simulink model "ssae_model"  (Simulink 7.3)
settings: Solver=ode3  StartTime=0.0  StopTime=2000.0  FixedStep=1  MaxStep=1  RelTol=1e-3
settings Model: Creator=alkis  LastModifiedBy=alkis
settings DataIOCC: MaxDataPoints=10000
settings DebuggingCC: SolverPrmCheckMsg=none

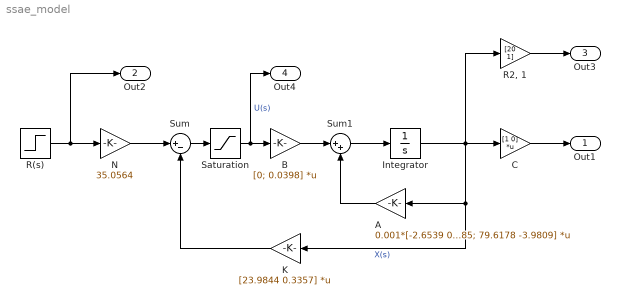
== system ssae_model ==
  A : Gain  Gain=0.001*[-2.6539 0.0885; 79.6178 -3.9809]  Multiplication=Matrix(K*u)  ParameterDataType=fixdt(1, 16)  ParameterScaling=2^0  OutDataType=fixdt(1, 16)  OutScaling=2^0
  B : Gain  Gain=[0; 0.0398]  Multiplication=Matrix(K*u)  ParameterDataType=fixdt(1, 16)  ParameterScaling=2^0  OutDataType=fixdt(1, 16)  OutScaling=2^0
  C : Gain  Gain=[1 0]  Multiplication=Matrix(K*u)  ParameterDataType=fixdt(1, 16)  ParameterScaling=2^0  OutDataType=fixdt(1, 16)  OutScaling=2^0
  Integrator : Integrator
  K : Gain  Gain=[23.9844 0.3357]  Multiplication=Matrix(K*u)  ParameterDataType=fixdt(1, 16)  ParameterScaling=2^0  OutDataType=fixdt(1, 16)  OutScaling=2^0
  N : Gain  Gain=35.0564  ParameterDataType=fixdt(1, 16)  ParameterScaling=2^0  OutDataType=fixdt(1, 16)  OutScaling=2^0
  R(s) : Step  Time=0  After=0.1  SampleTime=0
  "R2, 1" : Gain  Gain=[20 1]  ParameterDataType=fixdt(1, 16)  ParameterScaling=2^0  OutDataType=fixdt(1, 16)  OutScaling=2^0
  Saturation : Saturate  UpperLimit=3  LowerLimit=0  OutDataType=fixdt(1, 16)  OutScaling=2^0
  Sum : Sum  Inputs=|+-  OutDataType=fixdt(1, 16)  OutScaling=2^0
  Sum1 : Sum  Inputs=|++  OutDataType=fixdt(1, 16)  OutScaling=2^0
  Out1 : Outport  OutDataType=fixdt(1, 16)  OutScaling=2^0
  Out2 : Outport  Port=2  OutDataType=fixdt(1, 16)  OutScaling=2^0
  Out3 : Outport  Port=3  OutDataType=fixdt(1, 16)  OutScaling=2^0
  Out4 : Outport  Port=4  OutDataType=fixdt(1, 16)  OutScaling=2^0
  wires:
  R(s)/1 -> N/1, Out2/1
  N/1 -> Sum/1
  C/1 -> Out1/1
  Integrator/1 -> C/1, K/1, A/1, "R2, 1"/1  "X(s)"
  Sum/1 -> Saturation/1
  K/1 -> Sum/2
  Saturation/1 -> B/1, Out4/1  "U(s)"
  B/1 -> Sum1/1
  A/1 -> Sum1/2
  Sum1/1 -> Integrator/1
  "R2, 1"/1 -> Out3/1
